simulink model "Furuta_Simulink_Final"  (R2020a)
settings: Solver=FixedStepAuto  StartTime=0.0  StopTime=inf  RelTol=1e-3  EnableMultiTasking=on
values from neighbouring files (symbols this model uses):
  K = lqr(A,B,Q,R)    [System_Dynamics_And_LQR_Gains.m]
libraries: arduinolib x3
settings Model: SILPILModeSetting=veronly  ExtModeTrigDuration=2  Creator=Mohamed ibrahim  LastModifiedBy=DELL
settings OptimizationCC: EnhancedBackFolding=on  PassReuseOutputArgsAs=Individual arguments  ZeroExternalMemoryAtStartup=off  ZeroInternalMemoryAtStartup=off  MaxStackSize=64  OptimizeBlockOrder=speed  DifferentSizesBufferReuse=on  OptimizationCustomize=off  EfficientTunableParamExpr=on
settings DebuggingCC: ParameterTunabilityLossMsg=error  SFMachineParentedDataDiag=error
settings HardwareCC: ProdBitPerInt=16  ProdBitPerPointer=16  ProdBitPerSizeT=16  ProdBitPerPtrDiffT=16  ProdLargestAtomicFloat=None  ProdWordSize=8  ProdHWDeviceType=Atmel->AVR
settings SFSimCC: MATLABDynamicMemAlloc=off
settings RTWCC: SystemTargetFile=ert.tlc  HardwareBoard=Arduino Mega 2560  TLCOptions=-aInlineSetEventsForThisBaseRateFcn=TLC_FALSE -aSuppressMultiTaskScheduler=TLC_FALSE -aRateBasedStepFcn=1  TemplateMakefile=ert_default_tmf  Toolchain=Arduino AVR  BuildConfiguration=Faster Runs
settings CodeAppCC: ForceParamTrailComments=on  IgnoreCustomStorageClasses=off  OperatorAnnotations=on  SimulinkDataObjDesc=on  SFDataObjDesc=on  InsertBlockDesc=on
settings ERTTargetCC: SupportContinuousTime=on  SupportVariableSizeSignals=on  ExtModeStaticAllocSize=2048

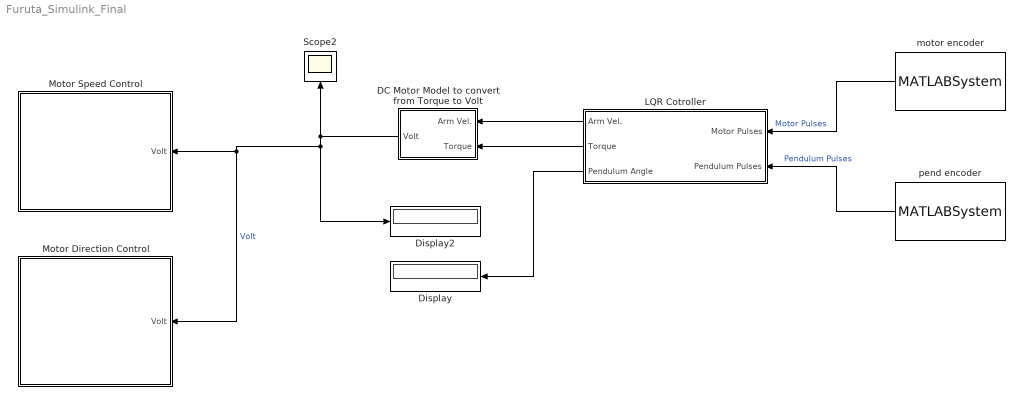
== system Furuta_Simulink_Final ==
  DC Motor Model to convert from Torque to Volt : Subsystem
  Display : Display
  Display2 : Display
  LQR Cotroller : Subsystem
  Motor Direction Control : Subsystem
  Motor Speed Control : Subsystem
  Scope2 : Scope
  motor encoder : MATLABSystem  System=Encoder_arduino  Encoder=0  PinA=2  PinB=3  SampleTime=0.01
      mask Type: Encoder_arduino
      mask Display:
      | disp('Encoder');
      | port_label('output',1,'y');
  pend encoder : MATLABSystem  System=Encoder_arduino  Encoder=1  PinA=18  PinB=19  SampleTime=0.01
      mask Type: Encoder_arduino
      mask Display:
      | disp('Encoder');
      | port_label('output',1,'y');
  wires:
  DC Motor Model to convert from Torque to Volt/1(Volt) -> Display2/1, Motor Speed Control/1(Volt), Motor Direction Control/1(Volt), Scope2/1  "Volt"
  motor encoder/1 -> LQR Cotroller/1(Motor Pulses)  "Motor Pulses"
  pend encoder/1 -> LQR Cotroller/2(Pendulum Pulses)  "Pendulum Pulses"
  LQR Cotroller/1(Arm Vel.) -> DC Motor Model to convert from Torque to Volt/1(Arm Vel.)
  LQR Cotroller/2(Torque) -> DC Motor Model to convert from Torque to Volt/2(Torque)
  LQR Cotroller/3(Pendulum Angle) -> Display/1

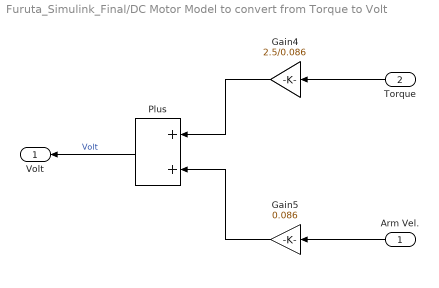
== system Furuta_Simulink_Final/DC Motor Model to convert from Torque to Volt ==
  Arm Vel. : Inport
  Torque : Inport  Port=2
  Gain4 : Gain  Gain=2.5/0.086
  Gain5 : Gain  Gain=0.086
  Plus : Sum
  Volt : Outport
  wires:
  Gain4/1 -> Plus/1
  Gain5/1 -> Plus/2
  Plus/1 -> Volt/1  "Volt"
  Arm Vel./1 -> Gain5/1
  Torque/1 -> Gain4/1

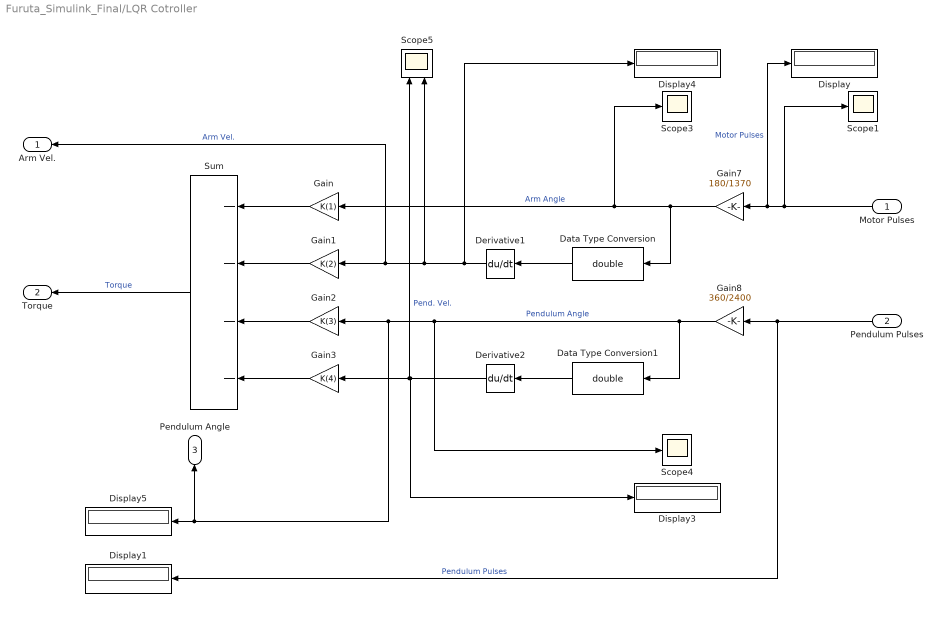
== system Furuta_Simulink_Final/LQR Cotroller ==
  Motor Pulses : Inport
  Pendulum Pulses : Inport  Port=2
  Data Type Conversion : DataTypeConversion  OutDataTypeStr=double
  Data Type Conversion1 : DataTypeConversion  OutDataTypeStr=double
  Derivative1 : Derivative
  Derivative2 : Derivative
  Display{,1,3..5} (5 alike) : Display
  Gain : Gain  Gain=K(1)
  Gain1 : Gain  Gain=K(2)
  Gain2 : Gain  Gain=K(3)
  Gain3 : Gain  Gain=K(4)
  Gain7 : Gain  Gain=180/1370
  Gain8 : Gain  Gain=360/2400
  Scope1 : Scope
  Scope3 : Scope
  Scope4 : Scope
  Scope5 : Scope  NumInputPorts=2
  Sum : Sum  Inputs=----
  Arm Vel. : Outport
  Torque : Outport  Port=2
  Pendulum Angle : Outport  Port=3
  wires:
  Gain3/1 -> Sum/4
  Gain7/1 -> Data Type Conversion/1, Gain/1, Scope3/1  "Arm Angle"
  Motor Pulses/1 -> Scope1/1, Display/1, Gain7/1  "Motor Pulses"
  Gain8/1 -> Data Type Conversion1/1, Scope4/1, Display5/1, Pendulum Angle/1, Gain2/1  "Pendulum Angle"
  Derivative1/1 -> Display4/1, Arm Vel./1, Gain1/1, Scope5/2  "Arm Vel."
  Gain1/1 -> Sum/2
  Gain/1 -> Sum/1
  Gain2/1 -> Sum/3
  Pendulum Pulses/1 -> Display1/1, Gain8/1  "Pendulum Pulses"
  Derivative2/1 -> Scope5/1, Gain3/1, Display3/1  "Pend. Vel."
  Data Type Conversion1/1 -> Derivative2/1
  Data Type Conversion/1 -> Derivative1/1
  Sum/1 -> Torque/1  "Torque"

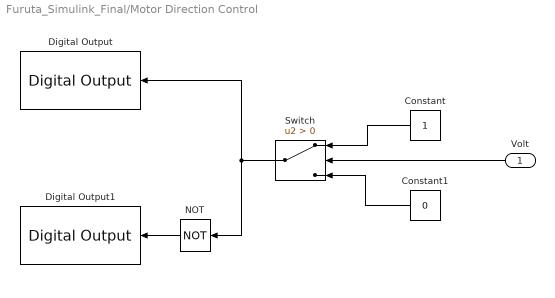
== system Furuta_Simulink_Final/Motor Direction Control ==
  Volt : Inport
  Constant : Constant
  Constant1 : Constant  Value=0
  Digital Output : arduinolib/Digital Output  pinNumber=22  Direction=output  blockPlatform=arduino
  Digital Output1 : arduinolib/Digital Output  pinNumber=23  Direction=output  blockPlatform=arduino
  NOT : Logic  Operator=NOT  IconShape=distinctive  AllPortsSameDT=off  OutDataTypeStr=boolean
  Switch : Switch  Criteria=u2 > Threshold
  wires:
  Constant/1 -> Switch/1
  Volt/1 -> Switch/2
  Switch/1 -> Digital Output/1, NOT/1
  NOT/1 -> Digital Output1/1
  Constant1/1 -> Switch/3

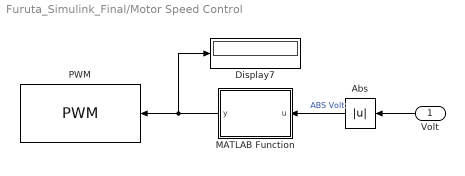
== system Furuta_Simulink_Final/Motor Speed Control ==
  Volt : Inport
  Abs : Abs
  Display7 : Display
  MATLAB Function : MATLAB Function  TreatAsAtomicUnit=on
  PWM : arduinolib/PWM  pinNumber=9  frequencyType=Default  desiredFrequency=490.2  achievableFrequency=490.2
  wires:
  Volt/1 -> Abs/1
  Abs/1 -> MATLAB Function/1(u)  "ABS Volt"
  MATLAB Function/1(y) -> Display7/1, PWM/1

== matlab function Furuta_Simulink_Final/Motor Speed Control/MATLAB Function ==
  data: u input; y output
function y = fcn(u)
x = u;
if x > 255
    x = 255;
else
    x = u + 128;
end
y = x;
